simulink model "OpenLoop1"  (Simulink 9.1)
settings: Solver=ode4  StartTime=0.0  StopTime=60*5  RelTol=1e-3  EnableMultiTasking=on
undefined symbols (not defined in the file or in its folder): MIO, National_Instruments, PCI
libraries: sldrtlib x2
settings Model: Creator=Houska  LastModifiedBy=melab2  SimulationMode=external  ExtModeTrigDuration=10000
settings DataIOCC: LimitDataPoints=on  SignalLoggingSaveFormat=ModelDataLogs  SaveOutput=off  SaveTime=off  SignalLoggingName=logsOut
settings OptimizationCC: InitFltsAndDblsToZero=on  LifeSpan=auto
settings DebuggingCC: SaveWithParameterizedLinksMsg=none  SignalResolutionControl=TryResolveAllWithWarning  MultiTaskDSMMsg=warning  MultiTaskCondExecSysMsg=none  FcnCallInpInsideContextMsg=warning
settings HardwareCC: ProdBitPerPointer=64  ProdBitPerSizeT=64  ProdBitPerPtrDiffT=64  ProdLargestAtomicFloat=Float  ProdIntDivRoundTo=Zero  ProdEndianess=LittleEndian  ProdWordSize=64  ProdHWDeviceType=Intel->x86-64 (Windows64)
settings RTWCC: SystemTargetFile=sldrt.tlc  TemplateMakefile=sldrt.tmf  Description=Simulink Desktop Real-Time  RTWCompilerOptimization=on
settings CodeAppCC: MaxIdLength=95
settings SimulinkDesktopRealTimeCC: TargetPreCompLibLocation=C:\Program Files\MATLAB\R2018a\toolbox\sldrt\lib\win64  TargetLangStandard=C89/C90 (ANSI)  ModelReferenceCompliant=off  CompOptLevelCompliant=off  SupportVariableSizeSignals=off
settings ConfigComp: CovSFcnEnable=off

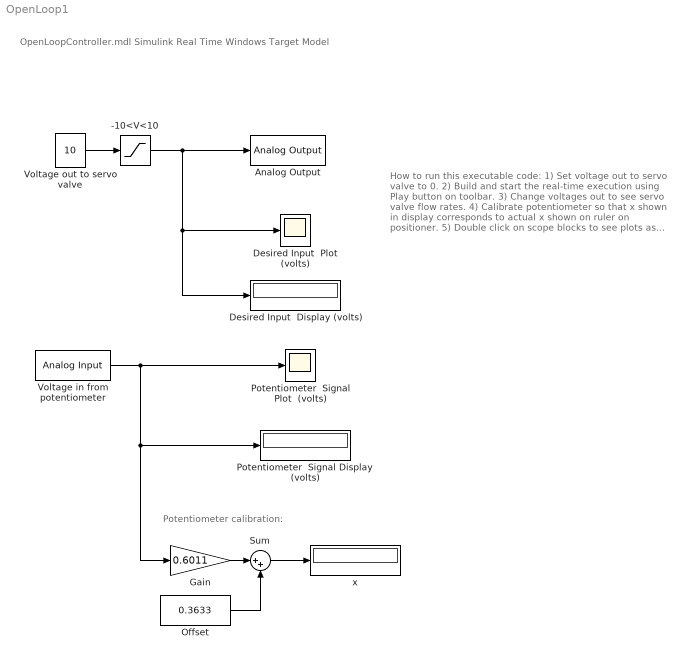
== system OpenLoop1 ==
  note: Potentiometer calibration:
  note: OpenLoopController.mdl
      | Simulink Real Time Windows Target Model
  note: How to run this executable code:
      |
      | 1) Set voltage out to servo valve to 0.
      |
      | 2) Build and start the real-time execution using
      |     Play button on toolbar.
      |
      | 3) Change voltages out to see servo valve
      |     flow rates.
      |
      | 4) Calibrate potentiometer so that x shown
      |     in display corresponds to actual x shown
      |     on ruler on positioner.
      |
      | 5) Double click on scope blocks to see plots
      |     as needed.
  -10<V<10 : Saturate  UpperLimit=10  LowerLimit=-10
  Analog Output : sldrtlib/Analog Output  SampleTime=1e-2  MaxMissedTicks=10  ShowMissedTicks=off  YieldWhenWaiting=off  DrvName=National_Instruments/PCI-MIO-16E-4  DrvAddress=4294967295  DrvOptions=[0 0 0 0 0]  Channels=1  RangeMode=1  VoltRange=1  InitialValue=0  FinalValue=0
      settings: AttributesFormatString=National Instruments\nPCI-MIO-16E-4 [auto]  SourceProductName=Simulink Desktop Real-Time
  Desired Input  Display (volts) : Display
  Desired Input  Plot (volts) : Scope
  Gain : Gain  Gain=0.6011
  Offset : Constant  Value=0.3633
  Potentiometer  Signal Display  (volts) : Display
  Potentiometer  Signal Plot  (volts) : Scope
  Sum : Sum  Inputs=|++
  Voltage in from potentiometer : sldrtlib/Analog Input  SampleTime=1e-2  MaxMissedTicks=10  ShowMissedTicks=off  YieldWhenWaiting=off  DrvName=National_Instruments/PCI-MIO-16E-4  DrvAddress=4294967295  DrvOptions=[0 0 0 0 0]  Channels=2  RangeMode=1  VoltRange=1  DataType=1
      settings: AttributesFormatString=National Instruments\nPCI-MIO-16E-4 [auto]  SourceProductName=Simulink Desktop Real-Time
  Voltage out to servo valve : Constant  Value=10
  x : Display
  wires:
  Voltage in from potentiometer/1 -> Potentiometer  Signal Plot  (volts)/1, Gain/1, Potentiometer  Signal Display  (volts)/1
  Voltage out to servo valve/1 -> -10<V<10/1
  Offset/1 -> Sum/2
  Gain/1 -> Sum/1
  Sum/1 -> x/1
  -10<V<10/1 -> Analog Output/1, Desired Input  Display (volts)/1, Desired Input  Plot (volts)/1
